simulink model "dc_motor_23b"  (R2023b)
settings: Solver=VariableStepAuto  StartTime=0.0  StopTime=10.0  RelTol=1e-3
undefined symbols (not defined in the file): b, J, K, L, R
settings Model: Creator=Harish  LastModifiedBy=Harish
settings RTWCC: GPUComputeCapability=5.0

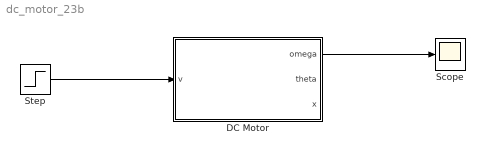
== system dc_motor_23b ==
  DC Motor : Subsystem
  Scope : Scope
  Step : Step  SampleTime=0
  wires:
  Step/1 -> DC Motor/1(v)
  DC Motor/1(omega) -> Scope/1

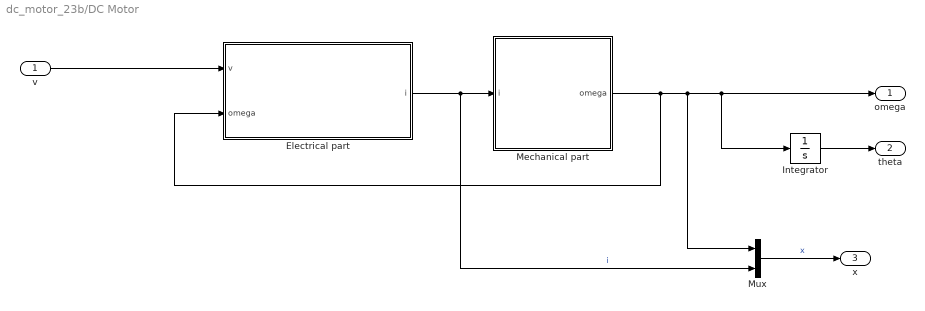
== system dc_motor_23b/DC Motor ==
  v : Inport
  "Electrical part " : Subsystem
  Integrator : Integrator
  Mechanical part : Subsystem
  Mux : Mux  Inputs=2
  omega : Outport
  theta : Outport  Port=2
  x : Outport  Port=3
  wires:
  "Electrical part "/1(i) -> Mux/2, Mechanical part/1(i)  "i"
  Mechanical part/1(omega) -> Mux/1, Integrator/1, omega/1, "Electrical part "/2(omega)
  v/1 -> "Electrical part "/1(v)
  Integrator/1 -> theta/1
  Mux/1 -> x/1  "x"

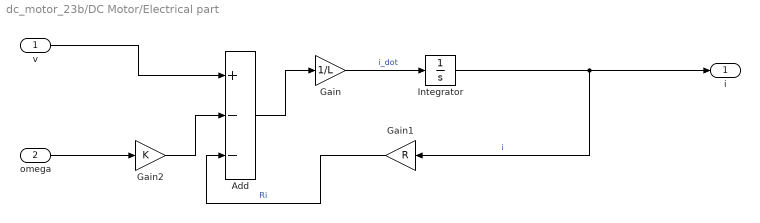
== system dc_motor_23b/DC Motor/Electrical part  ==
  v : Inport
  omega : Inport  Port=2
  Add : Sum  Inputs=+--
  Gain : Gain  Gain=1/L
  Gain1 : Gain  Gain=R
  Gain2 : Gain  Gain=K
  Integrator : Integrator
  i : Outport
  wires:
  Add/1 -> Gain/1
  Integrator/1 -> i/1, Gain1/1  "i"
  Gain1/1 -> Add/3  "Ri"
  v/1 -> Add/1
  Gain2/1 -> Add/2
  Gain/1 -> Integrator/1  "i_dot"
  omega/1 -> Gain2/1

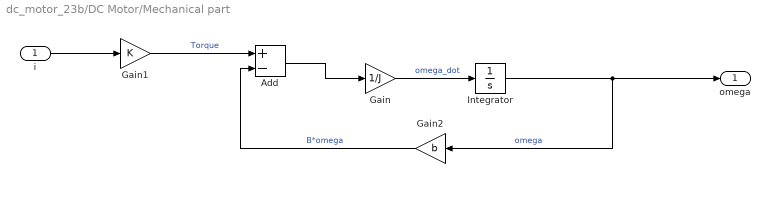
== system dc_motor_23b/DC Motor/Mechanical part ==
  i : Inport
  Add : Sum  Inputs=+-
  Gain : Gain  Gain=1/J
  Gain1 : Gain  Gain=K
  Gain2 : Gain  Gain=b
  Integrator : Integrator
  omega : Outport
  wires:
  Add/1 -> Gain/1
  Integrator/1 -> omega/1, Gain2/1  "omega"
  Gain2/1 -> Add/2  "B*omega"
  i/1 -> Gain1/1
  Gain/1 -> Integrator/1  "omega_dot"
  Gain1/1 -> Add/1  "Torque"
